simulink model "TrafficLight_Task"  (R2021a)
settings: Solver=FixedStepDiscrete  StartTime=0.0  StopTime=10.0  RelTol=1e-3
settings Model: Creator=Mohamed Elomda  LastModifiedBy=Mohamed Elomda
settings OptimizationCC: DefaultParameterBehavior=Inlined  EnhancedBackFolding=on  PassReuseOutputArgsAs=Individual arguments  ZeroExternalMemoryAtStartup=off  ZeroInternalMemoryAtStartup=off  OptimizeBlockOrder=speed  DifferentSizesBufferReuse=on  OptimizationCustomize=off  EfficientTunableParamExpr=on
settings DebuggingCC: UnderspecifiedInitializationDetection=Classic  MergeDetectMultiDrivingBlocksExec=none  ParameterTunabilityLossMsg=error
settings ModelReferenceCC: PropagateSignalLabelsOutOfModel=off
settings SFSimCC: MATLABDynamicMemAlloc=off
settings RTWCC: SystemTargetFile=ert.tlc  GenCodeOnly=on  TemplateMakefile=ert_default_tmf  GenerateReport=on  LaunchReport=on
settings CodeAppCC: ForceParamTrailComments=on  IgnoreCustomStorageClasses=off  OperatorAnnotations=on  SimulinkDataObjDesc=on  SFDataObjDesc=on  InsertBlockDesc=on
settings ERTTargetCC: TargetLangStandard=C99 (ISO)  GenerateSampleERTMain=on  InlinedParameterPlacement=NonHierarchical  ERTCustomFileTemplate=example_file_process.tlc

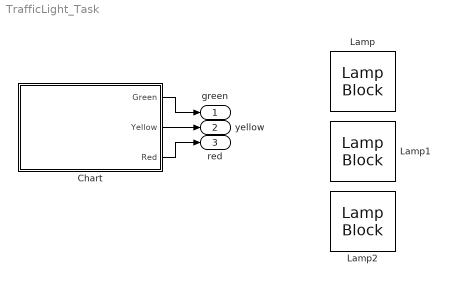
== system TrafficLight_Task ==
  Chart : Stateflow chart  TreatAsAtomicUnit=on
  Lamp : LampBlock  LabelPosition=Hide
  Lamp1 : LampBlock  LabelPosition=Hide
  Lamp2 : LampBlock  LabelPosition=Hide
  green : Outport  SignalName=Green
  yellow : Outport  Port=2  SignalName=Yellow
  red : Outport  Port=3  SignalName=Red
  wires:
  Chart/1(Green) -> green/1
  Chart/3(Red) -> red/1
  Chart/2(Yellow) -> yellow/1

== stateflow chart TrafficLight_Task/Chart ==
  state Stop
    entry:
    Red = 1;
    Yellow = 0;
    Green = 0;
  state PrepareToStop
    entry:
    Red = 0;
    Yellow = 1;
    Green = 0;
  state Go
    entry:
    Red = 0;
    Yellow = 0;
    Green = 1;
  (default) -> Stop
  Go -> Stop : after(3,sec)
  Stop -> PrepareToStop : after(3,sec)
  PrepareToStop -> Go : after(3,sec)
  data: Green output =0; Yellow output =0; Red output =0
